simulink library "afl"  (Simulink 7.0)
undefined symbols (not defined in the file or in its folder): ENUM_FAULTSTATE_FAIL, ENUM_FAULTSTATE_PASS, FALSE, TRUE
settings Model: Creator=GTR  LastModifiedBy=R00T

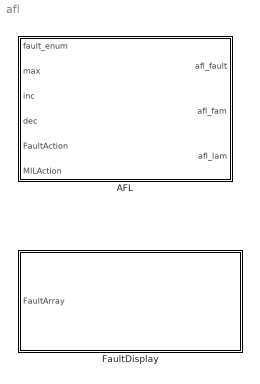
== system afl ==
  AFL : Subsystem
  FaultDisplay : Subsystem  TreatAsAtomicUnit=on

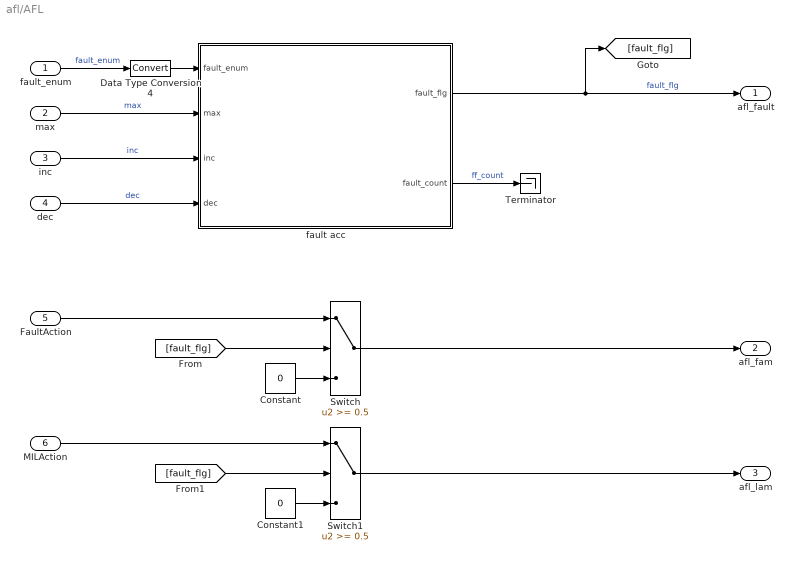
== system afl/AFL ==
  fault_enum : Inport
  max : Inport  Port=2
  inc : Inport  Port=3
  dec : Inport  Port=4
  FaultAction : Inport  Port=5
  MILAction : Inport  Port=6
  Constant : Constant  Value=0  OutDataTypeMode=uint16
  Constant1 : Constant  Value=0  OutDataTypeMode=uint16
  Data Type Conversion4 : DataTypeConversion  OutDataTypeMode=uint8
  Switch : Switch  Threshold=0.5
  Switch1 : Switch  Threshold=0.5
  Terminator : Terminator
  fault acc : Stateflow chart  TreatAsAtomicUnit=on
  afl_fault : Outport
  afl_fam : Outport  Port=2
  afl_lam : Outport  Port=3
  wires:
  Switch1/1 -> afl_lam/1
  MILAction/1 -> Switch1/1
  Switch/1 -> afl_fam/1
  FaultAction/1 -> Switch/1
  Constant/1 -> Switch/3
  fault acc/2(fault_count) -> Terminator/1  "ff_count"
  inc/1 -> fault acc/3(inc)  "inc"
  fault acc/1(fault_flg) -> [fault_flg], afl_fault/1  "fault_flg"
  dec/1 -> fault acc/4(dec)  "dec"
  fault_enum/1 -> Data Type Conversion4/1  "fault_enum"
  Data Type Conversion4/1 -> fault acc/1(fault_enum)
  max/1 -> fault acc/2(max)  "max"
  [fault_flg] -> Switch/2
  Constant1/1 -> Switch1/3
  [fault_flg] -> Switch1/2

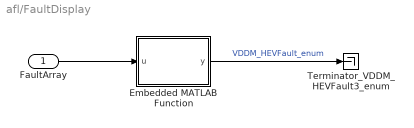
== system afl/FaultDisplay ==
  FaultArray : Inport  OutDataType=fixdt(1, 16)  OutScaling=2^0
  Embedded MATLAB Function : Stateflow chart
  Terminator_VDDM_HEVFault3_enum : Terminator
  wires:
  Embedded MATLAB Function/1(y) -> Terminator_VDDM_HEVFault3_enum/1  "VDDM_HEVFault_enum"
  FaultArray/1 -> Embedded MATLAB Function/1(u)

== stateflow chart AFL/fault acc ==
  (junction 5) -> (junction 9)
  (junction 3) -> (junction 10) [order 1] : [fault_enum==ENUM_FAULTSTATE_FAIL]
  (junction 12) -> (junction 13) : {count-=dec;}
  (junction 14) -> (junction 15) : {count = 0;
      | fault_flg=FALSE;}
  (junction 16) -> (junction 17) : {count = max;
      | fault_flg = TRUE;}
  (junction 4) -> (junction 5) [order 3]
  (junction 9) -> (junction 6) : {fault_count = count;}
  (junction 7) -> (junction 4)
  (default) -> (junction 8)
  (junction 8) -> (junction 3)
  (junction 10) -> (junction 11) : {count+=inc;}
  (junction 3) -> (junction 12) [order 2] : [fault_enum==ENUM_FAULTSTATE_PASS]
  (junction 13) -> (junction 7)
  (junction 11) -> (junction 7)
  (junction 3) -> (junction 7) [order 3]
  (junction 4) -> (junction 14) [order 2] : [count <= 0]
  (junction 4) -> (junction 16) [order 1] : [count >= max]
  (junction 15) -> (junction 5)
  (junction 17) -> (junction 5)
  data: fault_enum input uint8; max input uint16; inc input uint8; dec input uint8; fault_flg output boolean =0; fault_count output int16; count local int16 =0; TRUE parameter boolean; FALSE parameter boolean; ENUM_FAULTSTATE_PASS parameter uint8; ENUM_FAULTSTATE_FAIL parameter uint8

== matlab function FaultDisplay/Embedded MATLAB Function ==
  data: u input double; y output double
function y = fcn(u)
MAX_LENGTH=8;
y=uint8(zeros(MAX_LENGTH,1));
%y = array_sorted(1:MAX_LENGTH);
indexCurrent=1;
for i=1:length(u)
 if u(i)~=0 && indexCurrent<=MAX_LENGTH
     y(indexCurrent)=uint8(i);
     indexCurrent=indexCurrent+1;
 end
end
